simulink model "Punto_3_y_4"  (R2023a)
settings: Solver=VariableStepAuto  StartTime=0  StopTime=7.02  RelTol=1e-3
libraries: simulink x10
settings Model: Creator=laura  LastModifiedBy=laura

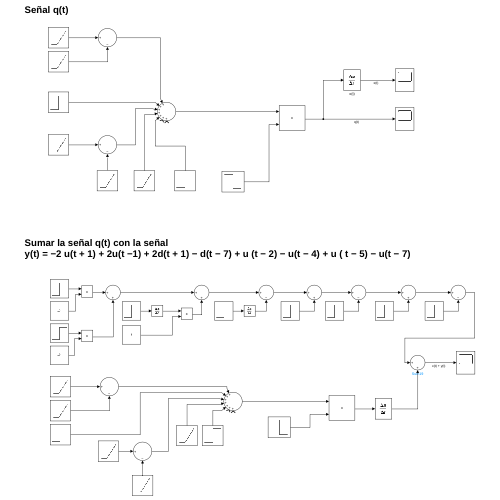
[thumbnail: Simulink's stored preview of the top-level diagram]
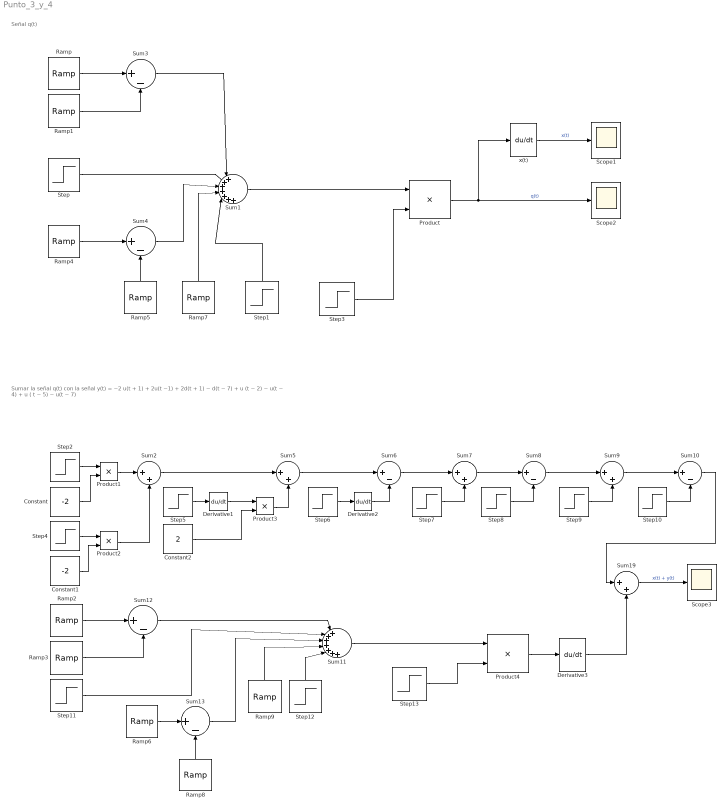
== system Punto_3_y_4 ==
  note: Sumar la señal q(t) con la señal
      | y(t) = −2 u(t + 1) + 2u(t −1) + 2d(t + 1) − d(t − 7) + u (t − 2) − u(t − 4) + u ( t − 5) − u(t − 7)
  note: Señal q(t)
  Constant : Constant  Value=-2
  Constant1 : Constant  Value=-2
  Constant2 : Constant  Value=2
  Derivative1 : Derivative
  Derivative2 : Derivative
  Derivative3 : Derivative
  Product{,1..4} (5 alike) : Product
  Ramp : simulink/Sources/Ramp  slope=2  start=0  InitialOutput=0
  Ramp1 : simulink/Sources/Ramp  slope=2  start=1  InitialOutput=0
  Ramp2 : simulink/Sources/Ramp  slope=2  start=0  InitialOutput=0
  Ramp3 : simulink/Sources/Ramp  slope=2  start=1  InitialOutput=0
  Ramp4 : simulink/Sources/Ramp  slope=-1  start=2  InitialOutput=0
  Ramp5 : simulink/Sources/Ramp  slope=-1  start=4  InitialOutput=0
  Ramp6 : simulink/Sources/Ramp  slope=-1  start=2  InitialOutput=0
  Ramp7 : simulink/Sources/Ramp  slope=-1  start=5  InitialOutput=0
  Ramp8 : simulink/Sources/Ramp  slope=-1  start=4  InitialOutput=0
  Ramp9 : simulink/Sources/Ramp  slope=-1  start=5  InitialOutput=0
  Scope1 : Scope
  Scope2 : Scope
  Scope3 : Scope
  Step : Step  Time=2  SampleTime=0
  Step1 : Step  Time=7  SampleTime=0
  Step10 : Step  Time=8  SampleTime=0
  Step11 : Step  Time=2  SampleTime=0
  Step12 : Step  Time=7  SampleTime=0
  Step13 : Step  Time=7  Before=1  After=0  SampleTime=0
  Step2 : Step  Time=0  SampleTime=0
  Step3 : Step  Time=7  Before=1  After=0  SampleTime=0
  Step4 : Step  Time=2  SampleTime=0
  Step5 : Step  Time=0  SampleTime=0
  Step6 : Step  Time=8  SampleTime=0
  Step7 : Step  Time=3  SampleTime=0
  Step8 : Step  Time=5  SampleTime=0
  Step9 : Step  Time=6  SampleTime=0
  Sum1 : Sum  Inputs=|+++++++
  Sum{3..4,6,8,10,12..13} (7 alike) : Sum  Inputs=|+-
  Sum11 : Sum  Inputs=|+++++++
  Sum{2,5,7,9,19} (5 alike) : Sum  Inputs=|++
  x(t) : Derivative
  wires:
  Ramp/1 -> Sum3/1
  Ramp1/1 -> Sum3/2
  Sum3/1 -> Sum1/1
  Ramp4/1 -> Sum4/1
  Step/1 -> Sum1/2
  Sum4/1 -> Sum1/3
  Ramp5/1 -> Sum4/2
  Ramp7/1 -> Sum1/4
  Step1/1 -> Sum1/5
  Product/1 -> Scope2/1, x(t)/1  "q(t)"
  Sum1/1 -> Product/1
  Step3/1 -> Product/2
  x(t)/1 -> Scope1/1  "x(t)"
  Derivative1/1 -> Product3/1
  Product2/1 -> Sum2/2
  Step6/1 -> Derivative2/1
  Step7/1 -> Sum7/2
  Constant2/1 -> Product3/2
  Step4/1 -> Product2/1
  Step9/1 -> Sum9/2
  Product3/1 -> Sum5/2
  Sum6/1 -> Sum7/1
  Product1/1 -> Sum2/1
  Sum2/1 -> Sum5/1
  Sum9/1 -> Sum10/1
  Step2/1 -> Product1/1
  Step5/1 -> Derivative1/1
  Sum5/1 -> Sum6/1
  Constant/1 -> Product1/2
  Sum7/1 -> Sum8/1
  Sum19/1 -> Scope3/1  "x(t) + y(t)"
  Sum8/1 -> Sum9/1
  Step10/1 -> Sum10/2
  Constant1/1 -> Product2/2
  Sum10/1 -> Sum19/1
  Step8/1 -> Sum8/2
  Derivative2/1 -> Sum6/2
  Ramp6/1 -> Sum13/1
  Ramp8/1 -> Sum13/2
  Sum11/1 -> Product4/1
  Step12/1 -> Sum11/5
  Product4/1 -> Derivative3/1
  Ramp9/1 -> Sum11/4
  Sum12/1 -> Sum11/1
  Sum13/1 -> Sum11/3
  Step11/1 -> Sum11/2
  Ramp2/1 -> Sum12/1
  Ramp3/1 -> Sum12/2
  Step13/1 -> Product4/2
  Derivative3/1 -> Sum19/2
